simulink model "sistema_1a_ordem_analogico_e_digital"  (R2016b)
settings: Solver=VariableStepAuto  StartTime=0.0  StopTime=50  RelTol=1e-3
settings Model: Creator=fernandopassold  LastModifiedBy=fernandopassold

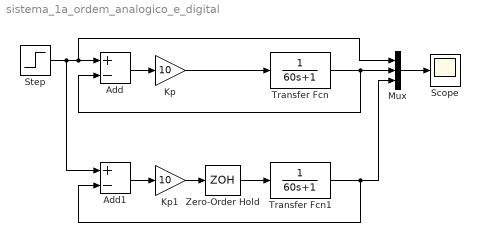
== system sistema_1a_ordem_analogico_e_digital ==
  Add : Sum  Inputs=+-
  Add1 : Sum  Inputs=+-
  Kp : Gain  Gain=10
  Kp1 : Gain  Gain=10
  Mux : Mux  Inputs=3
  Scope : Scope
  Step : Step  SampleTime=0
  Transfer Fcn : TransferFcn  Denominator=[60 1]
  Transfer Fcn1 : TransferFcn  Denominator=[60 1]
  Zero-Order Hold : ZeroOrderHold  SampleTime=5
  wires:
  Add/1 -> Kp/1
  Mux/1 -> Scope/1
  Transfer Fcn/1 -> Add/2, Mux/2
  Kp/1 -> Transfer Fcn/1
  Step/1 -> Add1/1, Mux/1, Add/1
  Add1/1 -> Kp1/1
  Transfer Fcn1/1 -> Add1/2, Mux/3
  Kp1/1 -> Zero-Order Hold/1
  Zero-Order Hold/1 -> Transfer Fcn1/1
